simulink model "PID_Controller"  (R2015b)
settings: Solver=VariableStepAuto  StartTime=0.0  StopTime=10.0  RelTol=1e-3
values from neighbouring files (symbols this model uses):
  c = 500e-6    (= 0.0005)    [Class_11_28_16_Example.m]    (also in Ellipsoid.m = 3; MTRE3710_Assignment_17.m = (f-32)*5/9)
  J = vertcat(JV,JW)    [Symbolic_Robot_Project.m]
undefined symbols (not defined in the file or in its folder): k0, khw
libraries: simulink x1
settings Model: Creator=Jacques-Ezechiel  LastModifiedBy=Jacques-Ezechiel

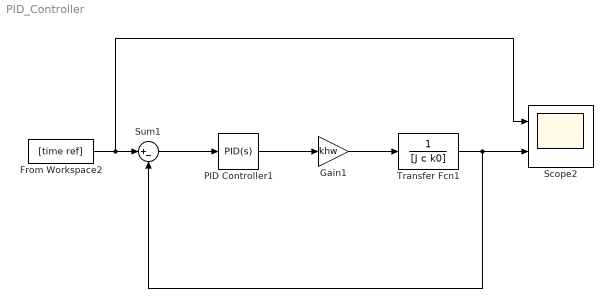
== system PID_Controller ==
  From Workspace2 : FromWorkspace  VariableName=[time ref]  SampleTime=0  OutputAfterFinalValue=Setting to zero
  Gain1 : Gain  Gain=khw
  PID Controller1 : simulink/Continuous/PID Controller  Controller=PID  TimeDomain=Continuous-time  SampleTime=-1  IntegratorMethod=Forward Euler  FilterMethod=Forward Euler  Form=Parallel  UseFilter=on  ControllerParametersSource=internal  P=8  I=30  D=5  N=100  InitialConditionSource=internal  InitialConditionForIntegrator=0  InitialConditionForFilter=0  ExternalReset=none  LimitOutput=off  UpperSaturationLimit=inf  LowerSaturationLimit=-inf  LinearizeAsGain=on  AntiWindupMode=none  Kb=1  TrackingMode=off  Kt=1  PParamMin=[]  PParamMax=[]  IParamMin=[]  IParamMax=[]  DParamMin=[]  DParamMax=[]  NParamMin=[]  NParamMax=[]  KbParamMin=[]  KbParamMax=[]  KtParamMin=[]  KtParamMax=[]  POutMin=[]  POutMax=[]  IOutMin=[]  IOutMax=[]  DOutMin=[]  DOutMax=[]  NOutMin=[]  NOutMax=[]  KbOutMin=[]  KbOutMax=[]  KtOutMin=[]  KtOutMax=[]  IntegratorOutMin=[]  IntegratorOutMax=[]  FilterOutMin=[]  FilterOutMax=[]  SumOutMin=[]  SumOutMax=[]  SumI1OutMin=[]  SumI1OutMax=[]  SumI2OutMin=[]  SumI2OutMax=[]  SumI3OutMin=[]  SumI3OutMax=[]  SumDOutMin=[]  SumDOutMax=[]  SaturationOutMin=[]  SaturationOutMax=[]  IntegratorContinuousStateAttributes=''  IntegratorStateMustResolveToSignalObject=off  IntegratorRTWStateStorageClass=Auto  FilterContinuousStateAttributes=''  FilterStateMustResolveToSignalObject=off  FilterRTWStateStorageClass=Auto  DifferentiatorICPrevScaledInput=0  DifferentiatorOutMin=[]  DifferentiatorOutMax=[]
  Scope2 : Scope  NumInputPorts=2
  Sum1 : Sum  Inputs=|+-
  Transfer Fcn1 : TransferFcn  Denominator=[J c k0]
  wires:
  Sum1/1 -> PID Controller1/1
  PID Controller1/1 -> Gain1/1
  Gain1/1 -> Transfer Fcn1/1
  Transfer Fcn1/1 -> Scope2/2, Sum1/2
  From Workspace2/1 -> Scope2/1, Sum1/1
